simulink model "BSCU_Brake_Mode_tmp"  (Simulink 8.4)
settings: Solver=ode45  StartTime=0.0  StopTime=10.0  RelTol=1e-3
undefined symbols (not defined in the file): LO, MANUAL, MAX, MED
settings Model: Creator=bourbouh  LastModifiedBy=hbourbou  CovSFcnEnable=on
settings DataIOCC: LimitDataPoints=off  SaveFormat=StructureWithTime  SignalLoggingSaveFormat=Dataset
settings OptimizationCC: ExpressionDepthLimit=128
settings DebuggingCC: UnderspecifiedInitializationDetection=Simplified  MergeDetectMultiDrivingBlocksExec=error  SolverPrmCheckMsg=none  FcnCallInpInsideContextMsg=EnableAllAsError  FrameProcessingCompatibilityMsg=error  StateNameClashWarn=none
settings HardwareCC: ProdBitPerPointer=64  ProdLargestAtomicFloat=Float  ProdIntDivRoundTo=Zero  ProdEndianess=LittleEndian  ProdHWDeviceType=Specified
settings ModelReferenceCC: PropagateSignalLabelsOutOfModel=on
settings GRTTargetCC: CombineOutputUpdateFcns=on  GRTInterface=off

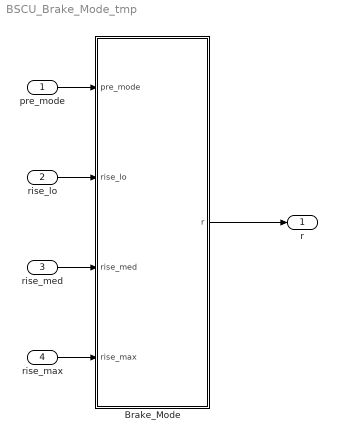
== system BSCU_Brake_Mode_tmp ==
  pre_mode : Inport
  rise_lo : Inport  Port=2
  rise_med : Inport  Port=3
  rise_max : Inport  Port=4
  Brake_Mode : Stateflow chart  TreatAsAtomicUnit=on
      settings: PermitHierarchicalResolution=ParametersOnly
  r : Outport
  wires:
  pre_mode/1 -> Brake_Mode/1(pre_mode)
  rise_lo/1 -> Brake_Mode/2(rise_lo)
  rise_med/1 -> Brake_Mode/3(rise_med)
  rise_max/1 -> Brake_Mode/4(rise_max)
  Brake_Mode/1(r) -> r/1

== stateflow chart Brake_Mode ==
  (default) -> (junction 12)
  (junction 12) -> (junction 13) [order 1] : [  ((pre_mode == LO) && rise_lo) || ...
      |    ((pre_mode == MED) && rise_med) || ...
      |    ((pre_mode == MAX) && rise_max)
      | ]
  (junction 12) -> (junction 14) [order 2]
  (junction 13) -> (junction 24) : {
      | r = MANUAL;
      | }
  (junction 14) -> (junction 15) [order 1] : [  (pre_mode != LO) && rise_lo ]
  (junction 14) -> (junction 16) [order 2]
  (junction 15) -> (junction 23) : {
      | r = LO;
      | }
  (junction 16) -> (junction 17) [order 1] : [ (pre_mode != MED) && rise_med ]
  (junction 16) -> (junction 18) [order 2]
  (junction 17) -> (junction 22) : {
      | r = MED;
      | }
  (junction 18) -> (junction 19) [order 1] : [ (pre_mode != MAX) && rise_max ]
  (junction 18) -> (junction 20) [order 2] : {
      | r = pre_mode;
      | }
  (junction 19) -> (junction 21) : {
      | r = MAX;
      | }
  (junction 21) -> (junction 20)
  (junction 22) -> (junction 21)
  (junction 23) -> (junction 22)
  (junction 24) -> (junction 23)
  (junction 20) -> (junction 25)
  data: pre_mode input int32; rise_lo input boolean; rise_med input boolean; rise_max input boolean; r output int32; MANUAL parameter int32 =1; LO parameter int32 =2; MED parameter int32 =3; MAX parameter int32 =4
